simulink model "Lab1_3"  (R2023a)
settings: Solver=ode45  StartTime=0.0  StopTime=10000/20e6  RelTol=1e-3  EnableMultiTasking=on
undefined symbols (not defined in the file): fdesignblkfcn, gcbh, xc7z020clg484, xlfda_numerator
libraries: hdlBasic x13, dspfdesign x1, hdlUtilities x1, hdlDSPIP x1, vmcUtilities x1
(part 1 of 3)
settings Model: Creator=danielm  LastModifiedBy=kodim
settings SolverCC: AlgebraicLoopSolver=TrustRegion
settings DataIOCC: LimitDataPoints=on  SaveFormat=Array  ReturnWorkspaceOutputs=off
settings OptimizationCC: LifeSpan=inf
settings DebuggingCC: UnderspecifiedInitializationDetection=Classic  MergeDetectMultiDrivingBlocksExec=none  SolverPrmCheckMsg=warning  UnconnectedInputMsg=warning  UnconnectedOutputMsg=warning  UnconnectedLineMsg=warning  SFUnexpectedBacktrackingDiag=warning  SFNoUnconditionalDefaultTransitionDiag=warning  SFExecutionAtInitializationDiag=none  ArithmeticOperatorsInVariantConditions=warning
settings HardwareCC: ProdBitPerPointer=32  ProdBitPerSizeT=32  ProdBitPerPtrDiffT=32  ProdLargestAtomicFloat=None  ProdIntDivRoundTo=Undefined  ProdEndianess=Unspecified  ProdWordSize=32  ProdHWDeviceType=32-bit Generic
settings ModelReferenceCC: EnableRefExpFcnMdlSchedulingChecks=on  PropagateSignalLabelsOutOfModel=off
settings SFSimCC: SimUseLocalCustomCode=off  CustomCodeUndefinedFunction=UseInterfaceOnly
settings RTWCC: RTWUseLocalCustomCode=off  DLArmComputeVersion=19.05
settings CodeAppCC: StateflowObjectComments=on
settings GRTTargetCC: TargetLangStandard=C89/C90 (ANSI)
settings ConfigComp: CovMetricSettings=dw  CovSaveCumulativeToWorkspaceVar=on  CovSaveSingleToWorkspaceVar=on  CovExternalEMLEnable=off  CovSFcnEnable=off

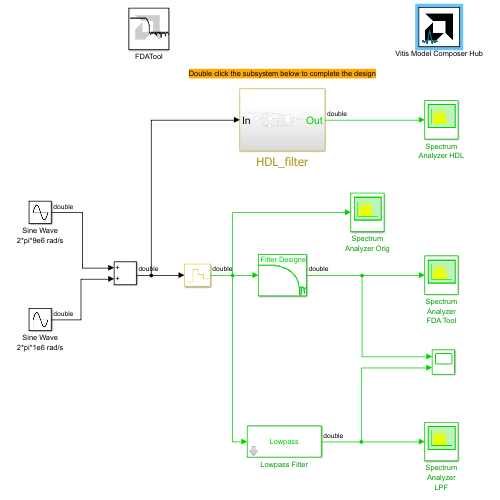
[thumbnail: Simulink's stored preview of the top-level diagram]
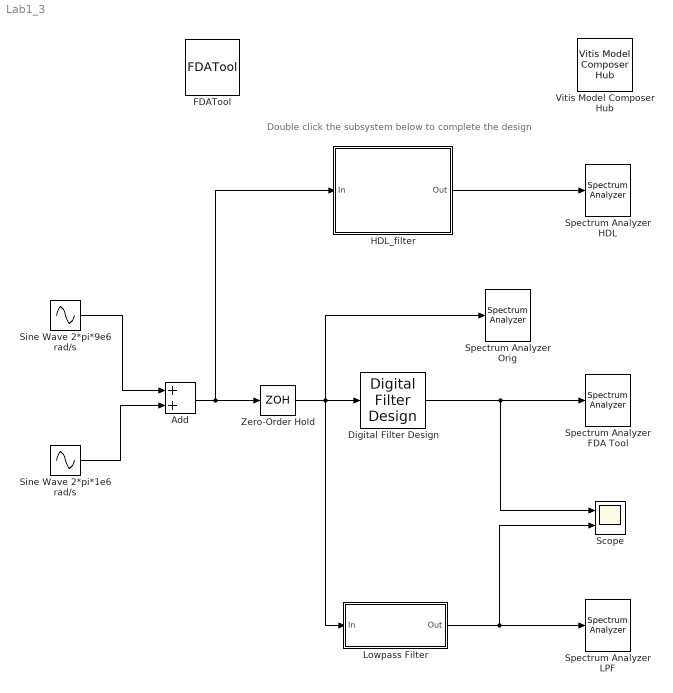
== system Lab1_3 ==
  note: Double click the subsystem below to complete the design
  Add : Sum
  Digital Filter Design : dspfdesign/Digital Filter Design  mwdsp_browser_bugfix_var=off
  FDATool : hdlUtilities/FDATool  block_type=fdatool
      settings: infoedit=FDATool
  HDL_filter : Subsystem
  Lowpass Filter : Subsystem  DialogController=fdesignblkfcn  InitFcn=fdesignblkfcn(gcbh, {'InitFcn'});  mask(Lowpass Filter){}
      mask help: Design a lowpass filter
      settings: CopyFcn=fdesignblkfcn(gcbh, {'CopyFcn'});
      mask Help: helpview(mapfilelocation('dsp'), 'dsplowpassfilter');
      mask Display: disp('Lowpass')
  Scope : Scope  NumInputPorts=2
  Sine Wave 2*pi*1e6 rad/s : Sin  Frequency=2*pi*1e6  SampleTime=0
  Sine Wave 2*pi*9e6 rad/s : Sin  Frequency=2*pi*9e6  SampleTime=0
  Spectrum Analyzer FDA Tool : SpectrumAnalyzer  WindowPosition=[863.000000,549.000000,576.000000,420.000000,]  ScopeFrameLocation=window  Method=Welch  SampleRate=20000000  AveragingMethod=Exponential  YLimits=[-188.67239893,47.37561541]  ChannelNames="[\"\"]"  DefaultConfigurationName=spbscopes.SpectrumAnalyzerBlockCfg
  Spectrum Analyzer LPF : SpectrumAnalyzer  WindowPosition=[161.000000,536.000000,576.000000,420.000000,]  ScopeFrameLocation=window  Method=Welch  SampleRate=20000000  AveragingMethod=Exponential  YLimits=[-188.98595007,47.39531461]  ChannelNames="[\"\"]"  DefaultConfigurationName=spbscopes.SpectrumAnalyzerBlockCfg
  "Spectrum Analyzer HDL " : SpectrumAnalyzer  WindowPosition=[856.000000,86.000000,568.000000,420.000000,]  ScopeFrameLocation=window  Method=Welch  SampleRate=20000000  AveragingMethod=Exponential  YLimits=[-189.91717723,47.51410963]  ChannelNames="[\"\"]"  DefaultConfigurationName=spbscopes.SpectrumAnalyzerBlockCfg
  Spectrum Analyzer Orig : SpectrumAnalyzer  WindowPosition=[114.000000,84.000000,584.000000,420.000000,]  ScopeFrameLocation=window  Method=Welch  SampleRate=20000000  AveragingMethod=Exponential  YLimits=[-154.28400242,43.53683553]  ChannelNames="[\"\"]"  DefaultConfigurationName=spbscopes.SpectrumAnalyzerBlockCfg
  Vitis Model Composer Hub : vmcUtilities/Vitis Model Composer Hub  Tag=genX  CodeGeneration=off  SubsystemName=HDL_filter  DUTSubsystemName=HDL_filter  CompilationType=HDLCompilation  ExportTypeV2=IP Catalog  TargetDirectory=D:/Files_ELEC_522/Assignments/Project1/Model_Composer_Tutorials/Lab1\ip\HDL_filter\src  exportDesign=off  analyzeDesign=on  validateDesignOnHw=off  ExportType=HDL  IpVendor=xilinx.com  IpLibrary=hls  IpVersion=1.0  IpHWLanguage=Verilog  AieCompilerOptions={}  AieSimulatorOptions={}  CreateTestbench=off  TestbenchStackSize=10  RunRtlSim=off  RunCSim=off  RunAieSim=off  AieSimTimeout=50000  RunAieSimProfiling=off  LaunchVitisAnalyzer=off  PlotOutput=off  RunX86Sim=off  X86SimTimeout=10  GenHwImage=off  GenLibadfXo=off  GenHwValidationCode=off  PlatformType=Not Specified  HwSystemType=Baremetal  HwValidationTarget=hw  ProjDevice=ZedBoard Zynq Evaluation and Development Kit (xc7z020clg484-1)  ProjDevicePart=xc7z020clg484-1  SamplePeriod=-1  ClockFrequency=200  DataPathParallelism=1  xilinxfamily=zynq  part=xc7z020  speed=-1  package=clg484  directory=D:/Files_ELEC_522/Assignments/Project1/Model_Composer_Tutorials/Lab1\ip\HDL_filter\src  testbench=on  incr_netlist=off  synthesis_tool=Vivado  clock_wrapper=Clock Enables  dbl_ovrd=According to Block Masks  dcm_input_clock_period=10  sysclk_period=8.33  simulink_period=1/220e6  eval_field=0  IPInfoJsonString="{\"HDLSubsystem\":{\"SubsystemName\":\"HDL_filter\",\"IPName\":\"hdl_filter\",\"IPLibrary\":\"VMC\",\"IPVendor\":\"User Company\",\"IPVersion\":\"1.0\",\"TargetDirectory\":\"D:/Files_ELEC_522/Assignments/Project1/Model_Composer_Tutorials/Lab1\",\"SubsystemDir\":\"D:/Files_ELEC_522/Assignments/Project1/Model_Composer_Tutorials/Lab1\\\\ip\\\\HDL_filter\"},\"SubsystemTag\":\"HDLNode\"}"  LogFileName=''  NThreads=4
  Zero-Order Hold : ZeroOrderHold  SampleTime=1/20e6
  wires:
  Sine Wave 2*pi*9e6 rad/s/1 -> Add/1
  Sine Wave 2*pi*1e6 rad/s/1 -> Add/2
  Digital Filter Design/1 -> Scope/1, Spectrum Analyzer FDA Tool/1
  Zero-Order Hold/1 -> Spectrum Analyzer Orig/1, Lowpass Filter/1(In), Digital Filter Design/1
  Lowpass Filter/1(Out) -> Scope/2, Spectrum Analyzer LPF/1
  Add/1 -> HDL_filter/1(In), Zero-Order Hold/1
  HDL_filter/1(Out) -> "Spectrum Analyzer HDL "/1
